simulink model "patient_model"  (R2021a)
settings: Solver=VariableStepAuto  StartTime=0.0  StopTime=10  RelTol=1e-3
settings Model: OrderedModelArguments=off  Creator=Surrin1999  LastModifiedBy=Surrin1999

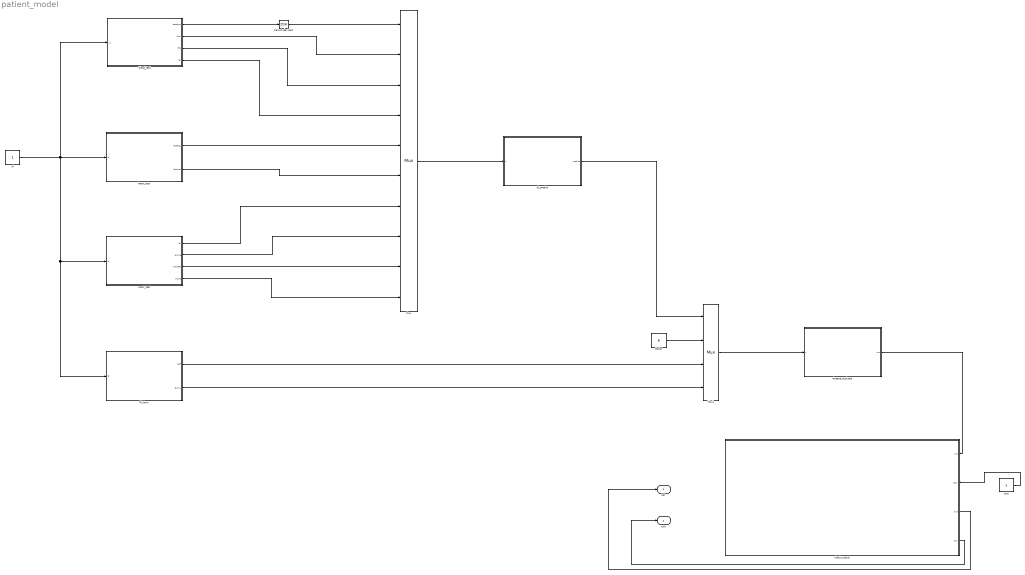
== system patient_model ==
  Mux : Mux  Inputs=10
  Mux1 : Mux
  Zero-Order Hold : ZeroOrderHold  SampleTime=5
  blood_test : Subsystem
  check_status : Stateflow chart  TreatAsAtomicUnit=on
      settings: PortSchema="{\"entries\":[{\"content\":{\"sides\":[{\"content\":{\"connectorIds\":[]},\"type\":\"ConnectorPlacement.EquallySpacedRectSide\",\"uuid\":\"e038a661-1200-4a0e-925f-654266734c7e\"},{\"content\":{\"connectorIds\":[\"In1\",\"In2\",\"Out1\",\"Out2\"],\"side\":\"RIGHT\"},\"type\":\"ConnectorPlacement.EquallySpacedRectSide\",\"uuid\":\"3ae57c8b-62f9-42d5-9b10-2ac471a64b9f\"},{\"content\":{\"connectorIds\":[],\"side\":\"TOP\"},\"type\":\"ConnectorPlacement.EquallySpacedRectSide\",\"uuid\":\"204d2454-9e03-4f19-9946-b136d7617ccc\"}]},\"type\":\"ConnectorPlacement.EquallySpacedConnector\",\"uuid\":\"205779e3-b196-48f4-a4e4-c5cd0711c9ad\"}],\"packageUris\":[\"http://schema.mathworks.com/mf0/Connector/R2020b\"],\"version\":\"1.0\"}"
  disease_evaluate : MATLAB Function  TreatAsAtomicUnit=on
  dl_predict : MATLAB Function  TreatAsAtomicUnit=on
  doctor : Constant  Value=8
  fill_form : Subsystem
  heart_test : Subsystem
  id : Constant
  sport_test : Subsystem
  stay : Constant
  pay : Outport
  exit : Outport  Port=2
  wires:
  blood_test/1(trestbps) -> Zero-Order Hold/1
  Zero-Order Hold/1 -> Mux/1
  blood_test/2(chol) -> Mux/2
  blood_test/3(fbs) -> Mux/3
  blood_test/4(ca) -> Mux/4
  heart_test/2(thalach) -> Mux/6
  sport_test/1(cp) -> Mux/7
  sport_test/2(exang) -> Mux/8
  sport_test/3(oldpeak) -> Mux/9
  sport_test/4(slope) -> Mux/10
  id/1 -> fill_form/1(id), sport_test/1(id), blood_test/1(id), heart_test/1(id)
  Mux/1 -> dl_predict/1(u)
  heart_test/1(restecg) -> Mux/5
  doctor/1 -> Mux1/2
  dl_predict/1(predict) -> Mux1/1
  fill_form/1(self) -> Mux1/3
  fill_form/2(family) -> Mux1/4
  Mux1/1 -> disease_evaluate/1(u)
  check_status/1(exit) -> pay/1
  check_status/2(pay) -> exit/1
  disease_evaluate/1(out) -> check_status/1(out)
  stay/1 -> check_status/2(stay)

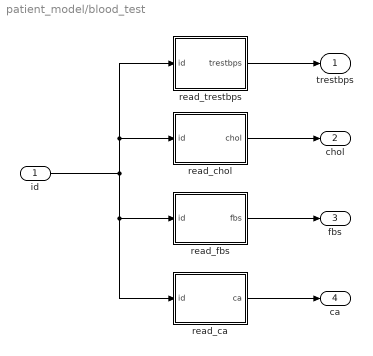
== system patient_model/blood_test ==
  id : Inport
  read_ca : MATLAB Function  TreatAsAtomicUnit=on
  read_chol : MATLAB Function  TreatAsAtomicUnit=on
  read_fbs : MATLAB Function  TreatAsAtomicUnit=on
  read_trestbps : MATLAB Function  TreatAsAtomicUnit=on
  trestbps : Outport
  chol : Outport  Port=2
  fbs : Outport  Port=3
  ca : Outport  Port=4
  wires:
  read_chol/1(chol) -> chol/1
  read_fbs/1(fbs) -> fbs/1
  read_trestbps/1(trestbps) -> trestbps/1
  id/1 -> read_chol/1(id), read_trestbps/1(id), read_ca/1(id), read_fbs/1(id)
  read_ca/1(ca) -> ca/1

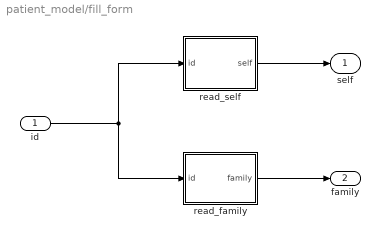
== system patient_model/fill_form ==
  id : Inport
  read_family : MATLAB Function  TreatAsAtomicUnit=on
  read_self : MATLAB Function  TreatAsAtomicUnit=on
  self : Outport
  family : Outport  Port=2
  wires:
  read_family/1(family) -> family/1
  read_self/1(self) -> self/1
  id/1 -> read_self/1(id), read_family/1(id)

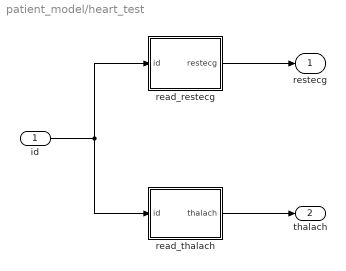
== system patient_model/heart_test ==
  id : Inport
  read_restecg : MATLAB Function  TreatAsAtomicUnit=on
  read_thalach : MATLAB Function  TreatAsAtomicUnit=on
  restecg : Outport
  thalach : Outport  Port=2
  wires:
  read_thalach/1(thalach) -> thalach/1
  read_restecg/1(restecg) -> restecg/1
  id/1 -> read_thalach/1(id), read_restecg/1(id)

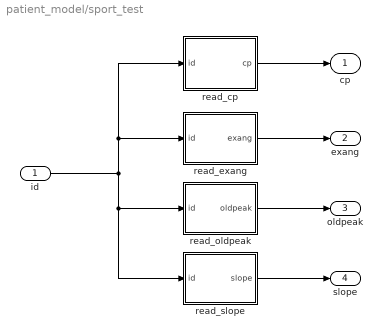
== system patient_model/sport_test ==
  id : Inport
  read_cp : MATLAB Function  TreatAsAtomicUnit=on
  read_exang : MATLAB Function  TreatAsAtomicUnit=on
  read_oldpeak : MATLAB Function  TreatAsAtomicUnit=on
  read_slope : MATLAB Function  TreatAsAtomicUnit=on
  cp : Outport
  exang : Outport  Port=2
  oldpeak : Outport  Port=3
  slope : Outport  Port=4
  wires:
  read_exang/1(exang) -> exang/1
  read_cp/1(cp) -> cp/1
  read_oldpeak/1(oldpeak) -> oldpeak/1
  read_slope/1(slope) -> slope/1
  id/1 -> read_exang/1(id), read_cp/1(id), read_slope/1(id), read_oldpeak/1(id)

== matlab function patient_model/fill_form/read_self ==
  data: id input; self output
function self = fcn(id)
  % result = 0;
  % coder.extrinsic('py.read_self.read');
  % result = py.read_self.read(id);
% self = result;
self = 0;

== matlab function patient_model/fill_form/read_family ==
  data: id input; family output
function family = fcn(id)
  % result = 0;
  % coder.extrinsic('py.read_family.read');
  % result = py.read_family.read(id);
% family = result;
family = 1;

== matlab function patient_model/dl_predict ==
  data: u input; predict output
function predict = fcn(u)
  result = 0;
  coder.extrinsic('py.dl.predict');
  result = double(py.dl.predict(u(1), u(2), u(3), u(4), u(5), u(6), u(7), u(8), u(9), u(10)));
predict = result;

== matlab function patient_model/disease_evaluate ==
  data: u input; out output
function out = fcn(u)
  predict = u(1);
  doctor = u(2);
  self = u(3);
  family = u(4);
  
  % set the weight respectively
  predict = predict * 0.25;
  doctor = doctor * 0.6;
  self = self * 0.1;
  family = family * 0.05;
  
  result = predict + doctor + self + family;
  disp(result);
  if result > 0.6
      out = 1;
  else
      out = 0;
  end

== stateflow chart patient_model/check_status ==
  (default) -> (junction 5)
  (junction 5) -> (junction 7) [order 1] : [out == 1]
  (junction 7) -> (junction 18) : {
      | pay = 1
      | }
  (junction 18) -> (junction 21) [order 1] : [stay == 1]
  (junction 21) -> (junction 15) : {
      | exit = 0;
      | }
  (junction 18) -> (junction 15) [order 2] : {
      | exit = 1;
      | }
  (junction 5) -> (junction 13) [order 2] : {
      | pay = 0;
      | exit = 1;
      | }
  (junction 13) -> (junction 15)
  data: out input; stay input; exit output; pay output

== matlab function patient_model/blood_test/read_chol ==
  data: id input; chol output
function chol = fcn(id)
  result = 0;
  coder.extrinsic('py.read_chol.read');
  result = py.read_chol.read(id);
chol = result;

== matlab function patient_model/blood_test/read_trestbps ==
  data: id input; trestbps output
function trestbps = fcn(id)
  result = 0;
  coder.extrinsic('py.read_trestbps.read');
  result = py.read_trestbps.read(id);
trestbps = result;

== matlab function patient_model/blood_test/read_fbs ==
  data: id input; fbs output
function fbs = fcn(id)
  result = 0;
  coder.extrinsic('py.read_fbs.read');
  result = py.read_fbs.read(id);
fbs = result;

== matlab function patient_model/heart_test/read_thalach ==
  data: id input; thalach output
function thalach = fcn(id)
  result = 0;
  coder.extrinsic('py.read_thalach.read');
  result = py.read_thalach.read(id);
thalach = result;

== matlab function patient_model/sport_test/read_cp ==
  data: id input; cp output
function cp = fcn(id)
  result = 0;
  coder.extrinsic('py.read_cp.read');
  result = py.read_cp.read(id);
cp = result;

== matlab function patient_model/heart_test/read_restecg ==
  data: id input; restecg output
function restecg = fcn(id)
  result = 0;
  coder.extrinsic('py.read_restecg.read');
  result = py.read_restecg.read(id);
restecg = result;

== matlab function patient_model/sport_test/read_exang ==
  data: id input; exang output
function exang = fcn(id)
  result = 0;
  coder.extrinsic('py.read_exang.read');
  result = py.read_exang.read(id);
exang = result;

== matlab function patient_model/sport_test/read_oldpeak ==
  data: id input; oldpeak output
function oldpeak = fcn(id)
  result = 0;
  coder.extrinsic('py.read_oldpeak.read');
  result = py.read_oldpeak.read(id);
oldpeak = result;

== matlab function patient_model/sport_test/read_slope ==
  data: id input; slope output
function slope = fcn(id)
  result = 0;
  coder.extrinsic('py.read_slope.read');
  result = py.read_slope.read(id);
slope = result;

== matlab function patient_model/blood_test/read_ca ==
  data: id input; ca output
function ca = fcn(id)
  result = 0;
  coder.extrinsic('py.read_ca.read');
  result = py.read_ca.read(id);
ca = result;
